simulink model "imsi"  (R2024b)
settings: Solver=VariableStepAuto  StartTime=0.0  StopTime=10.0  RelTol=1e-3
undefined symbols (not defined in the file): AI, AO, DI, DO
settings Model: Creator=HHI  LastModifiedBy=HHI

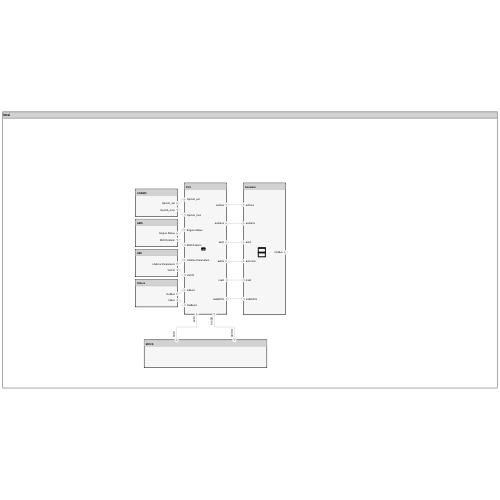
[thumbnail: Simulink's stored preview of the top-level diagram]
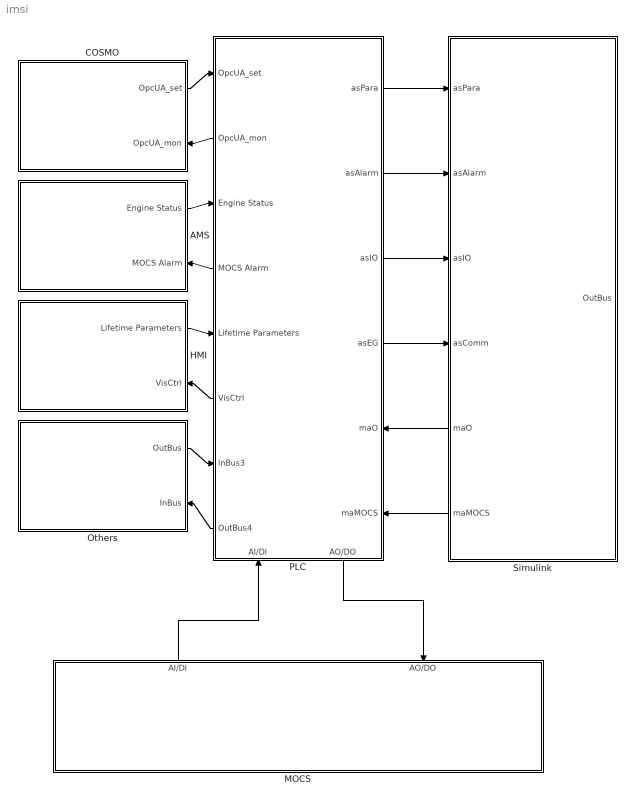
== system imsi ==
  AMS : Subsystem
      settings: PortSchema="{\"entries\":[{\"content\":{\"headerSize\":26,\"margin\":15,\"minimumSpacing\":25,\"sides\":[{\"content\":{},\"type\":\"ConnectorPlacement.EquallySpacedRectSide\",\"uuid\":\"599fdd01-6244-4eb5-99b9-9c0b863496cc\"},{\"content\":{\"connectorIds\":[\"Out1\",\"In1\"],\"side\":\"RIGHT\"},\"type\":\"ConnectorPlacement.EquallySpacedRectSide\",\"uuid\":\"8a9b10b5-2fcd-4fdc-9fbd-5ed5e98ed9ea\"},{\"content\":{\"side\":\"TOP\"},\"type\":\"ConnectorPlacement.EquallySpacedRectSide\",\"uuid\":\"a9917ffc-f231-45b7-935d-3896edcd0cfc\"}]},\"type\":\"ConnectorPlacement.EquallySpacedConnector\",\"uuid\":\"8a9c538d-2f59-4401-8937-d57b3a27c5f2\"}],\"packageUris\":[\"http://schema.mathworks.com/mf0/Connector/R2020b\"],\"version\":\"1.0\"}"
  COSMO : Subsystem
      settings: PortSchema="{\"entries\":[{\"content\":{\"headerSize\":26,\"margin\":15,\"minimumSpacing\":25,\"sides\":[{\"content\":{},\"type\":\"ConnectorPlacement.EquallySpacedRectSide\",\"uuid\":\"599fdd01-6244-4eb5-99b9-9c0b863496cc\"},{\"content\":{\"connectorIds\":[\"Out1\",\"In1\"],\"side\":\"RIGHT\"},\"type\":\"ConnectorPlacement.EquallySpacedRectSide\",\"uuid\":\"8a9b10b5-2fcd-4fdc-9fbd-5ed5e98ed9ea\"},{\"content\":{\"side\":\"TOP\"},\"type\":\"ConnectorPlacement.EquallySpacedRectSide\",\"uuid\":\"a9917ffc-f231-45b7-935d-3896edcd0cfc\"}]},\"type\":\"ConnectorPlacement.EquallySpacedConnector\",\"uuid\":\"8a9c538d-2f59-4401-8937-d57b3a27c5f2\"}],\"packageUris\":[\"http://schema.mathworks.com/mf0/Connector/R2020b\"],\"version\":\"1.0\"}"
  HMI : Subsystem
      settings: PortSchema="{\"entries\":[{\"content\":{\"headerSize\":26,\"margin\":15,\"minimumSpacing\":25,\"sides\":[{\"content\":{},\"type\":\"ConnectorPlacement.EquallySpacedRectSide\",\"uuid\":\"599fdd01-6244-4eb5-99b9-9c0b863496cc\"},{\"content\":{\"connectorIds\":[\"Out1\",\"In1\"],\"side\":\"RIGHT\"},\"type\":\"ConnectorPlacement.EquallySpacedRectSide\",\"uuid\":\"8a9b10b5-2fcd-4fdc-9fbd-5ed5e98ed9ea\"},{\"content\":{\"side\":\"TOP\"},\"type\":\"ConnectorPlacement.EquallySpacedRectSide\",\"uuid\":\"a9917ffc-f231-45b7-935d-3896edcd0cfc\"}]},\"type\":\"ConnectorPlacement.EquallySpacedConnector\",\"uuid\":\"8a9c538d-2f59-4401-8937-d57b3a27c5f2\"}],\"packageUris\":[\"http://schema.mathworks.com/mf0/Connector/R2020b\"],\"version\":\"1.0\"}"
  MOCS : Subsystem
      settings: PortSchema="{\"entries\":[{\"content\":{\"headerSize\":26,\"margin\":15,\"minimumSpacing\":25,\"sides\":[{\"content\":{},\"type\":\"ConnectorPlacement.EquallySpacedRectSide\",\"uuid\":\"599fdd01-6244-4eb5-99b9-9c0b863496cc\"},{\"content\":{\"side\":\"RIGHT\"},\"type\":\"ConnectorPlacement.EquallySpacedRectSide\",\"uuid\":\"8a9b10b5-2fcd-4fdc-9fbd-5ed5e98ed9ea\"},{\"content\":{\"connectorIds\":[\"Out1\",\"In1\"],\"side\":\"TOP\"},\"type\":\"ConnectorPlacement.EquallySpacedRectSide\",\"uuid\":\"a9917ffc-f231-45b7-935d-3896edcd0cfc\"}]},\"type\":\"ConnectorPlacement.EquallySpacedConnector\",\"uuid\":\"8a9c538d-2f59-4401-8937-d57b3a27c5f2\"}],\"packageUris\":[\"http://schema.mathworks.com/mf0/Connector/R2020b\"],\"version\":\"1.0\"}"
  Others : Subsystem
      settings: PortSchema="{\"entries\":[{\"content\":{\"headerSize\":26,\"margin\":15,\"minimumSpacing\":25,\"sides\":[{\"content\":{},\"type\":\"ConnectorPlacement.EquallySpacedRectSide\",\"uuid\":\"599fdd01-6244-4eb5-99b9-9c0b863496cc\"},{\"content\":{\"connectorIds\":[\"Out1\",\"In1\"],\"side\":\"RIGHT\"},\"type\":\"ConnectorPlacement.EquallySpacedRectSide\",\"uuid\":\"8a9b10b5-2fcd-4fdc-9fbd-5ed5e98ed9ea\"},{\"content\":{\"side\":\"TOP\"},\"type\":\"ConnectorPlacement.EquallySpacedRectSide\",\"uuid\":\"a9917ffc-f231-45b7-935d-3896edcd0cfc\"}]},\"type\":\"ConnectorPlacement.EquallySpacedConnector\",\"uuid\":\"8a9c538d-2f59-4401-8937-d57b3a27c5f2\"}],\"packageUris\":[\"http://schema.mathworks.com/mf0/Connector/R2020b\"],\"version\":\"1.0\"}"
  PLC : Subsystem
      settings: PortSchema="{\"entries\":[{\"content\":{\"headerSize\":26,\"margin\":15,\"minimumSpacing\":25,\"sides\":[{\"content\":{\"connectorIds\":[\"In1\",\"Out1\",\"In3\",\"Out6\",\"In4\",\"Out7\",\"In6\",\"Out8\"]},\"type\":\"ConnectorPlacement.EquallySpacedRectSide\",\"uuid\":\"599fdd01-6244-4eb5-99b9-9c0b863496cc\"},{\"content\":{\"connectorIds\":[\"Out9\",\"Out2\",\"Out3\",\"Out4\",\"In7\",\"In2\"],\"side\":\"RIGHT\"},\"type\":\"ConnectorPlacement.EquallySpacedRectSide\",\"uuid\":\"8a9b10b5-2fcd-4fdc-9fbd-5ed5e98ed9ea\"},{\"content\":{\"side\":\"TOP\"},\"type\":\"ConnectorPlacement.EquallySpacedRectSide\",\"uuid\":\"a9917ffc-f231-45b7-935d-3896edcd0cfc\"},{\"content\":{\"connectorIds\":[\"In5\",\"Out5\"],\"side\":\"BOTTOM\"},\"type\":\"ConnectorPlacement.EquallySpacedRectSide\",\"uuid\":\"1df8e97e-f77c-457a-9af7-e7e098554a93\"}]},\"type\":\"ConnectorPlacement.EquallySpacedConnector\",\"uuid\":\"8a9c538d-2f59-4401-8937-d57b3a27c5f2\"}],\"packageUris\":[\"http://schema.mathworks.com/mf0/Connector/R2020b\"],\"version\":\"1.0\"}"
  Simulink : Subsystem
      settings: PortSchema="{\"entries\":[{\"content\":{\"headerSize\":26,\"margin\":15,\"minimumSpacing\":25,\"sides\":[{\"content\":{\"connectorIds\":[\"In1\",\"In2\",\"In3\",\"In4\",\"Out3\",\"Out2\"]},\"type\":\"ConnectorPlacement.EquallySpacedRectSide\",\"uuid\":\"599fdd01-6244-4eb5-99b9-9c0b863496cc\"},{\"content\":{\"connectorIds\":[\"Out1\"],\"side\":\"RIGHT\"},\"type\":\"ConnectorPlacement.EquallySpacedRectSide\",\"uuid\":\"8a9b10b5-2fcd-4fdc-9fbd-5ed5e98ed9ea\"},{\"content\":{\"side\":\"TOP\"},\"type\":\"ConnectorPlacement.EquallySpacedRectSide\",\"uuid\":\"a9917ffc-f231-45b7-935d-3896edcd0cfc\"}]},\"type\":\"ConnectorPlacement.EquallySpacedConnector\",\"uuid\":\"8a9c538d-2f59-4401-8937-d57b3a27c5f2\"}],\"packageUris\":[\"http://schema.mathworks.com/mf0/Connector/R2020b\"],\"version\":\"1.0\"}"
  wires:
  COSMO/1(OpcUA_set) -> PLC/1(OpcUA_set)
  PLC/1(OpcUA_mon) -> COSMO/1(OpcUA_mon)
  AMS/1(Engine Status) -> PLC/3(Engine Status)
  PLC/6(MOCS Alarm) -> AMS/1(MOCS Alarm)
  HMI/1(Lifetime Parameters) -> PLC/4(Lifetime Parameters)
  PLC/7(VisCtrl) -> HMI/1(VisCtrl)
  Others/1(OutBus) -> PLC/6(InBus3)
  PLC/8(OutBus4) -> Others/1(InBus)
  PLC/9(asPara) -> Simulink/1(asPara)
  PLC/2(asAlarm) -> Simulink/2(asAlarm)
  PLC/3(asIO) -> Simulink/3(asIO)
  PLC/4(asEG) -> Simulink/4(asComm)
  Simulink/3(maO) -> PLC/7(maO)
  Simulink/2(maMOCS) -> PLC/2(maMOCS)
  PLC/5(AO/DO) -> MOCS/1(AO/DO)
  MOCS/1(AI/DI) -> PLC/5(AI/DI)

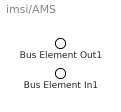
== system imsi/AMS ==
  Bus Element In1 : Inport  PortName=MOCS Alarm
  Bus Element Out1 : Outport  PortName=Engine Status

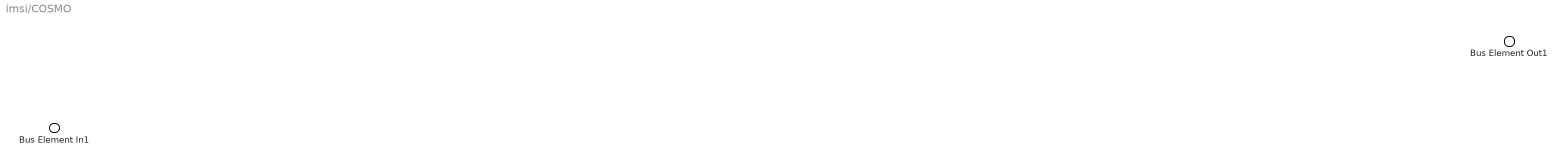
== system imsi/COSMO ==
  Bus Element In1 : Inport  PortName=OpcUA_mon
  Bus Element Out1 : Outport  PortName=OpcUA_set

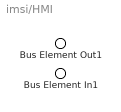
== system imsi/HMI ==
  Bus Element In1 : Inport  PortName=VisCtrl
  Bus Element Out1 : Outport  PortName=Lifetime Parameters

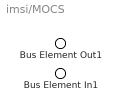
== system imsi/MOCS ==
  Bus Element In1 : Inport  PortName=AO/DO
  Bus Element Out1 : Outport  PortName=AI/DI

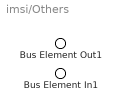
== system imsi/Others ==
  Bus Element In1 : Inport  PortName=InBus
  Bus Element Out1 : Outport  PortName=OutBus

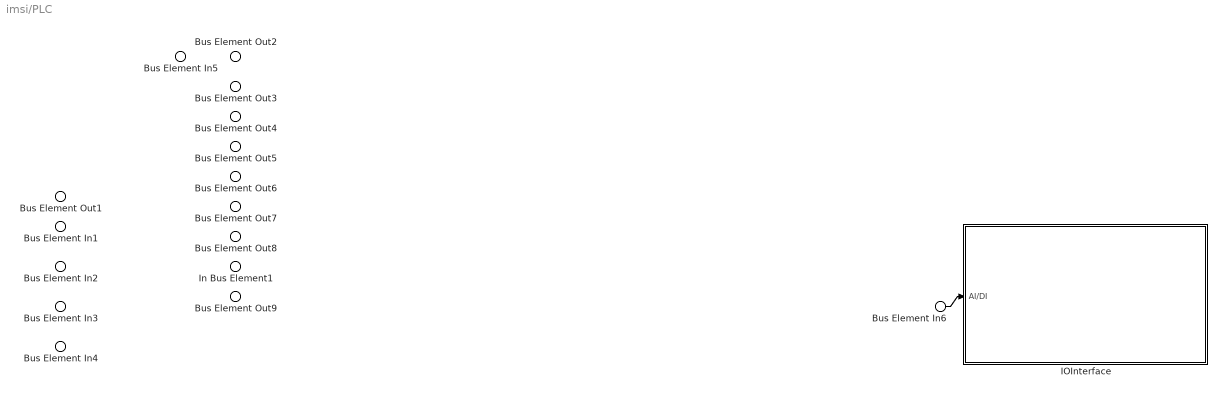
== system imsi/PLC ==
  Bus Element In1 : Inport  PortName=OpcUA_set
  Bus Element In5 : Inport  Port=2  PortName=maMOCS
  Bus Element In2 : Inport  Port=3  PortName=Engine Status
  Bus Element In3 : Inport  Port=4  PortName=Lifetime Parameters
  Bus Element In6 : Inport  Port=5  PortName=AI/DI
  Bus Element In4 : Inport  Port=6  PortName=InBus3
  In Bus Element1 : Inport  Port=7  PortName=maO
  IOInterface : Subsystem
      settings: PortSchema="{\"entries\":[{\"content\":{\"headerSize\":26,\"margin\":15,\"minimumSpacing\":25,\"sides\":[{\"content\":{\"connectorIds\":[\"In1\"]},\"type\":\"ConnectorPlacement.EquallySpacedRectSide\",\"uuid\":\"599fdd01-6244-4eb5-99b9-9c0b863496cc\"},{\"content\":{\"side\":\"RIGHT\"},\"type\":\"ConnectorPlacement.EquallySpacedRectSide\",\"uuid\":\"8a9b10b5-2fcd-4fdc-9fbd-5ed5e98ed9ea\"},{\"content\":{\"side\":\"TOP\"},\"type\":\"ConnectorPlacement.EquallySpacedRectSide\",\"uuid\":\"a9917ffc-f231-45b7-935d-3896edcd0cfc\"}]},\"type\":\"ConnectorPlacement.EquallySpacedConnector\",\"uuid\":\"8a9c538d-2f59-4401-8937-d57b3a27c5f2\"}],\"packageUris\":[\"http://schema.mathworks.com/mf0/Connector/R2020b\"],\"version\":\"1.0\"}"
  Bus Element Out2 : Outport  PortName=OpcUA_mon
  Bus Element Out6 : Outport  Port=2  PortName=asAlarm
  Bus Element Out7 : Outport  Port=3  PortName=asIO
  Bus Element Out8 : Outport  Port=4  PortName=asEG
  Bus Element Out9 : Outport  Port=5  PortName=AO/DO
  Bus Element Out3 : Outport  Port=6  PortName=MOCS Alarm
  Bus Element Out4 : Outport  Port=7  PortName=VisCtrl
  Bus Element Out5 : Outport  Port=8  PortName=OutBus4
  Bus Element Out1 : Outport  Port=9  PortName=asPara
  wires:
  Bus Element In6/1 -> IOInterface/1(AI/DI)

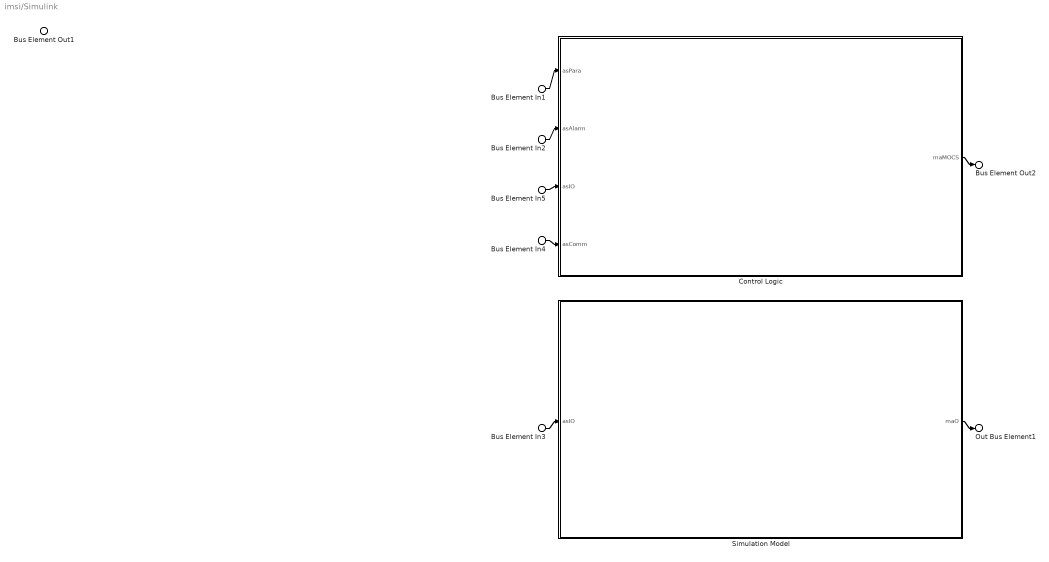
== system imsi/Simulink ==
  Bus Element In1 : Inport  PortName=asPara
  Bus Element In2 : Inport  Port=2  PortName=asAlarm
  Bus Element In3 : Inport  Port=3  PortName=asIO
  Bus Element In5 : Inport  Port=3  PortName=asIO
  Bus Element In4 : Inport  Port=4  PortName=asComm
  Control Logic : Subsystem
      settings: PortSchema="{\"entries\":[{\"content\":{\"headerSize\":26,\"margin\":15,\"minimumSpacing\":25,\"sides\":[{\"content\":{\"connectorIds\":[\"In1\",\"In2\",\"In3\",\"In4\"]},\"type\":\"ConnectorPlacement.EquallySpacedRectSide\",\"uuid\":\"599fdd01-6244-4eb5-99b9-9c0b863496cc\"},{\"content\":{\"connectorIds\":[\"Out1\"],\"side\":\"RIGHT\"},\"type\":\"ConnectorPlacement.EquallySpacedRectSide\",\"uuid\":\"8a9b10b5-2fcd-4fdc-9fbd-5ed5e98ed9ea\"},{\"content\":{\"side\":\"TOP\"},\"type\":\"ConnectorPlacement.EquallySpacedRectSide\",\"uuid\":\"a9917ffc-f231-45b7-935d-3896edcd0cfc\"}]},\"type\":\"ConnectorPlacement.EquallySpacedConnector\",\"uuid\":\"8a9c538d-2f59-4401-8937-d57b3a27c5f2\"}],\"packageUris\":[\"http://schema.mathworks.com/mf0/Connector/R2020b\"],\"version\":\"1.0\"}"
  Simulation Model : Subsystem
      settings: PortSchema="{\"entries\":[{\"content\":{\"headerSize\":26,\"margin\":15,\"minimumSpacing\":25,\"sides\":[{\"content\":{\"connectorIds\":[\"In1\"]},\"type\":\"ConnectorPlacement.EquallySpacedRectSide\",\"uuid\":\"599fdd01-6244-4eb5-99b9-9c0b863496cc\"},{\"content\":{\"connectorIds\":[\"Out1\"],\"side\":\"RIGHT\"},\"type\":\"ConnectorPlacement.EquallySpacedRectSide\",\"uuid\":\"8a9b10b5-2fcd-4fdc-9fbd-5ed5e98ed9ea\"},{\"content\":{\"side\":\"TOP\"},\"type\":\"ConnectorPlacement.EquallySpacedRectSide\",\"uuid\":\"a9917ffc-f231-45b7-935d-3896edcd0cfc\"}]},\"type\":\"ConnectorPlacement.EquallySpacedConnector\",\"uuid\":\"8a9c538d-2f59-4401-8937-d57b3a27c5f2\"}],\"packageUris\":[\"http://schema.mathworks.com/mf0/Connector/R2020b\"],\"version\":\"1.0\"}"
  Bus Element Out1 : Outport  PortName=OutBus
  Bus Element Out2 : Outport  Port=2  PortName=maMOCS
  Out Bus Element1 : Outport  Port=3  PortName=maO
  wires:
  Bus Element In1/1 -> Control Logic/1(asPara)
  Bus Element In2/1 -> Control Logic/2(asAlarm)
  Bus Element In3/1 -> Simulation Model/1(asIO)
  Bus Element In4/1 -> Control Logic/4(asComm)
  Bus Element In5/1 -> Control Logic/3(asIO)
  Simulation Model/1(maO) -> Out Bus Element1/1
  Control Logic/1(maMOCS) -> Bus Element Out2/1

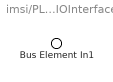
== system imsi/PLC/IOInterface ==
  Bus Element In1 : Inport  PortName=AI/DI

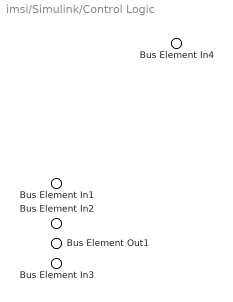
== system imsi/Simulink/Control Logic ==
  Bus Element In1 : Inport  PortName=asPara
  Bus Element In2 : Inport  Port=2  PortName=asAlarm
  Bus Element In4 : Inport  Port=3  PortName=asIO
  Bus Element In3 : Inport  Port=4  PortName=asComm
  Bus Element Out1 : Outport  PortName=maMOCS

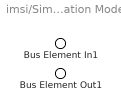
== system imsi/Simulink/Simulation Model ==
  Bus Element In1 : Inport  PortName=asIO
  Bus Element Out1 : Outport  PortName=maO
